simulink model "DC_Motor_2"  (R2016a)
settings: Solver=VariableStepAuto  StartTime=0.0  StopTime=3.0  RelTol=1e-3
settings Model: Creator=mmdclm  LastModifiedBy=Lara

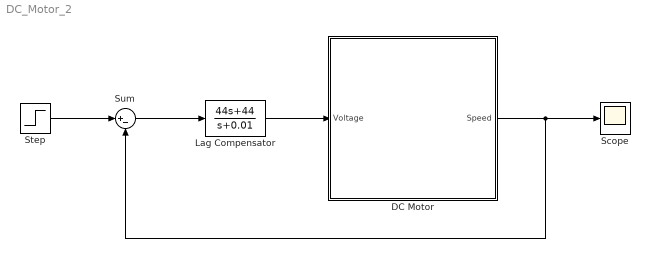
== system DC_Motor_2 ==
  "DC Motor " : Subsystem
  Lag Compensator : TransferFcn  Numerator=[44 44]  Denominator=[1 0.01]
  Scope : Scope
  Step : Step  Time=0  SampleTime=0
  Sum : Sum  Inputs=|+-
  wires:
  "DC Motor "/1("Speed ") -> Sum/2, Scope/1
  Step/1 -> Sum/1
  Lag Compensator/1 -> "DC Motor "/1(Voltage)
  Sum/1 -> Lag Compensator/1

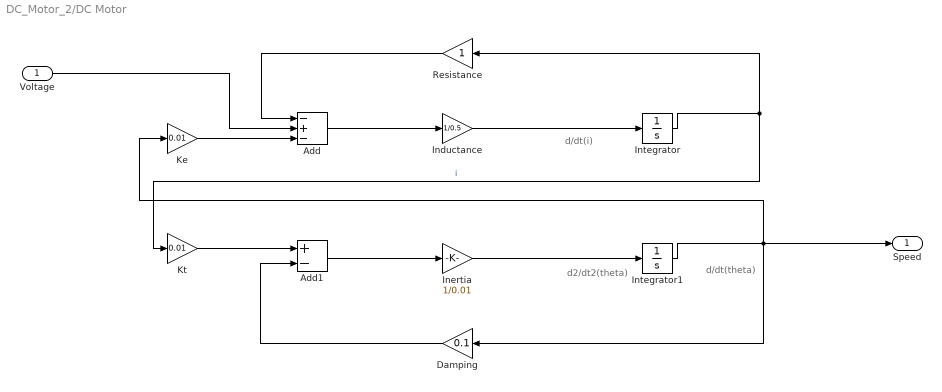
== system DC_Motor_2/DC Motor  ==
  note: d/dt(theta)
  note: d2/dt2(theta)
  note: d/dt(i)
  Voltage : Inport
  Add : Sum  Inputs=-+-
  Add1 : Sum  Inputs=+-
  Damping : Gain  Gain=0.1
  Inductance : Gain  Gain=1/0.5
  "Inertia " : Gain  Gain=1/0.01
  Integrator : Integrator
  Integrator1 : Integrator
  "Ke " : Gain  Gain=0.01
  "Kt " : Gain  Gain=0.01
  "Resistance " : Gain
  "Speed " : Outport
  wires:
  Voltage/1 -> Add/2
  Add/1 -> Inductance/1
  "Inertia "/1 -> Integrator1/1
  Add1/1 -> "Inertia "/1
  Integrator/1 -> "Kt "/1, "Resistance "/1  "i"
  "Ke "/1 -> Add/3
  Damping/1 -> Add1/2
  Inductance/1 -> Integrator/1
  "Kt "/1 -> Add1/1
  Integrator1/1 -> "Speed "/1, Damping/1, "Ke "/1
  "Resistance "/1 -> Add/1
